simulink model "ctrlSys_rl_env_test"  (R2025b)
settings: Solver=ode14x  StartTime=0.0  StopTime=100  FixedStep=Ts_local  RelTol=1e-4
model workspace (MAT data in the model file):
  CtrlChoice = "MPC_QP"
  FSI_max = [111.58614649; 109.244229433; 111.951462771]
  FSI_min = [3.65502707696; 3.64264743495; 3.42913459589]
  GateChoice = "linear"
  K1 = 1
  K2 = 1e-06
  Ncycle = 25
  SampEn_max = [0.399850516102; 0.373441099122; 0.45958437331]
  SampEn_min = [0.118794892672; 0.117721768048; 0.119599512992]
  fs = 5000
  m = 2
  rRatio = 0.2
values from neighbouring files (symbols this model uses):
  f = 50.0    [ctrlSys.sldd]
  Ts_ctrl = 0.1    [ctrlSys.sldd]
  Ts_local = 1.0E-5    [ctrlSys.sldd]
  Ts_meas = 0.005    [ctrlSys.sldd]
undefined symbols (not defined in the file or in its folder): R_rms, Rn_SNR, Ts_dist, v_lb, v_ub
libraries: ee_lib x13, simulink x5, nesl_utility x4, fl_lib x3, eeRmsMeasurement x3, rllib x1, slpidlib x1
settings Model: DataDictionary=ctrlSys.sldd  SimulationMode=accelerator  Creator=LYG  LastModifiedBy=i336
settings SolverCC: ZeroCrossControl=DisableAll
settings DataIOCC: SaveOutput=off  DSMLogging=off  SaveTime=off  ReturnWorkspaceOutputs=off

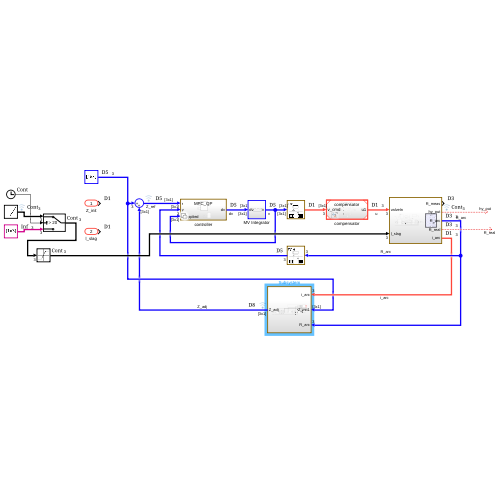
[thumbnail: Simulink's stored preview of the top-level diagram]
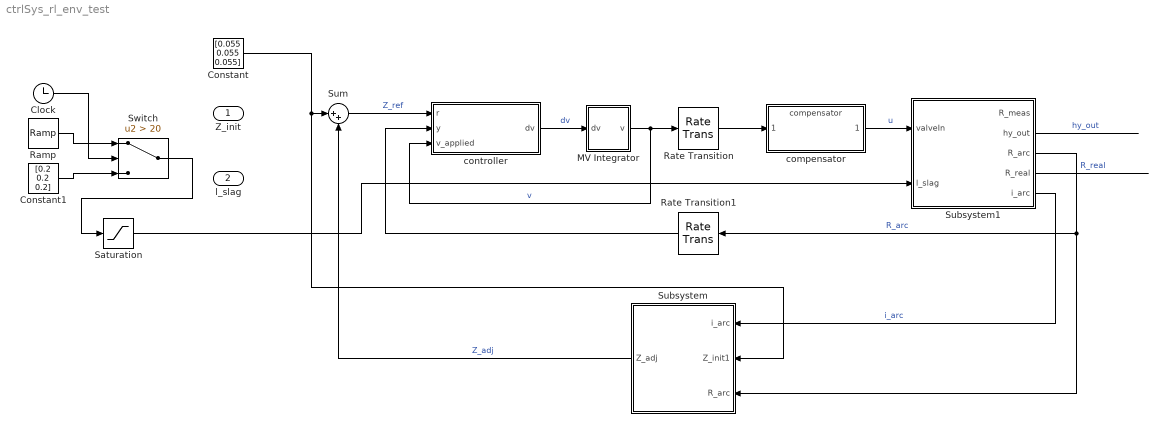
== system ctrlSys_rl_env_test ==
  Z_init : Inport  PortDimensions=3
  l_slag : Inport  Port=2  PortDimensions=3
  Clock : Clock
  Constant : Constant  Value=[0.055 0.055 0.055]  SampleTime=Ts_ctrl
  Constant1 : Constant  Value=[0.2 0.2 0.2]
  MV Integrator : Subsystem
  Ramp : simulink/Sources/Ramp  slope=(0.21 - 0.165) / (600 - 120)  start=[120 120 120]  InitialOutput=0.165
  Rate Transition : RateTransition  OutPortSampleTime=Ts_local
  Rate Transition1 : RateTransition  OutPortSampleTime=Ts_ctrl
  Saturation : Saturate  UpperLimit=0.21  LowerLimit=0
  Subsystem : Subsystem
  Subsystem1 : Subsystem
  Sum : Sum  Inputs=|++
  Switch : Switch  Criteria=u2 > Threshold  Threshold=20  SaturateOnIntegerOverflow=off  InputSameDT=off
  compensator : ModelReference  ModelNameDialog=compensator.slx  SimulationMode=Normal  ModelReferenceVersion=1.24
  controller : Subsystem  Variant=on
  wires:
  Rate Transition/1 -> compensator/1
  compensator/1 -> Subsystem1/1(valveIn)  "u"
  Subsystem1/3(R_arc) -> Subsystem/3(R_arc), Rate Transition1/1  "R_arc"
  Subsystem1/4(R_real) -> ?  "R_real"
  Rate Transition1/1 -> controller/2(y)
  MV Integrator/1(v) -> controller/3(v_applied), Rate Transition/1  "v"
  controller/1(dv) -> MV Integrator/1(dv)  "dv"
  Sum/1 -> controller/1(r)  "Z_ref"
  Subsystem/1(Z_adj) -> Sum/2  "Z_adj"
  Subsystem1/5(i_arc) -> Subsystem/1(i_arc)  "i_arc"
  Subsystem1/2(hy_out) -> ?  "hy_out"
  Constant/1 -> Subsystem/2(Z_init1), Sum/1
  Saturation/1 -> Subsystem1/2(l_slag)
  Clock/1 -> Switch/2
  Ramp/1 -> Switch/1
  Constant1/1 -> Switch/3
  Switch/1 -> Saturation/1

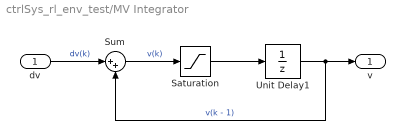
== system ctrlSys_rl_env_test/MV Integrator ==
  dv : Inport
  Saturation : Saturate  UpperLimit=v_ub  LowerLimit=v_lb
  Sum : Sum  Inputs=|++
  Unit Delay1 : UnitDelay  SampleTime=-1  HasFrameUpgradeWarning=on
  v : Outport
  wires:
  Saturation/1 -> Unit Delay1/1
  Unit Delay1/1 -> v/1, Sum/2  "v(k - 1)"
  dv/1 -> Sum/1  "dv(k)"
  Sum/1 -> Saturation/1  "v(k)"

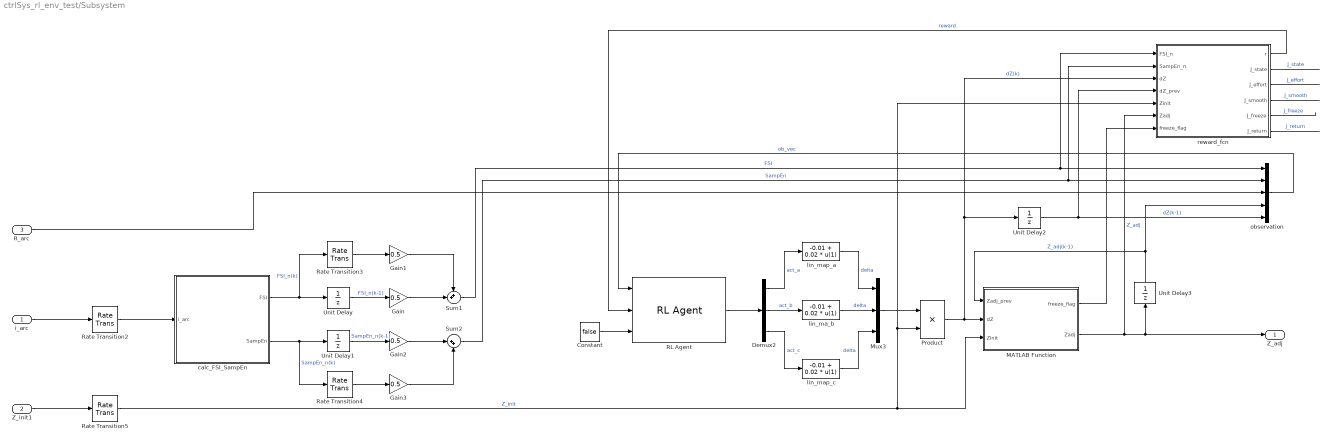
== system ctrlSys_rl_env_test/Subsystem ==
  i_arc : Inport  SampleTime=Ts_local
  Z_init1 : Inport  Port=2  PortDimensions=[3 1]  SampleTime=Ts_ctrl
  R_arc : Inport  Port=3  PortDimensions=3  SampleTime=Ts_meas
  Constant : Constant  Value=false
  Demux2 : Demux  Outputs=3
  Gain{,1..3} (4 alike) : Gain  Gain=0.5
  MATLAB Function : MATLAB Function  TreatAsAtomicUnit=on
  Mux3 : Mux  Inputs=3
  Product : Product
  RL Agent : rllib/RL Agent  Agent=agent  ExternalActionAsInput=off  ProvideLastAction=off  ProvideCumRwd=off  TreatAsDirectFeedthrough=on  UseStrictObservationDataTypes=off
  Rate Transition2 : RateTransition  OutPortSampleTime=1 / fs
  Rate Transition3 : RateTransition  OutPortSampleTime=Ncycle * (1 / f)
  Rate Transition4 : RateTransition  OutPortSampleTime=Ncycle * (1 / f)
  Rate Transition5 : RateTransition  OutPortSampleTime=Ts_sup
  Sum1 : Sum  Inputs=++|
  Sum2 : Sum  Inputs=|++
  Unit Delay : UnitDelay  SampleTime=Ncycle * (1 / f)  HasFrameUpgradeWarning=on
  Unit Delay1 : UnitDelay  SampleTime=Ncycle * (1 / f)  HasFrameUpgradeWarning=on
  Unit Delay2 : UnitDelay  SampleTime=-1  HasFrameUpgradeWarning=on
  Unit Delay3 : UnitDelay  SampleTime=-1  HasFrameUpgradeWarning=on
  calc_FSI_SampEn : MATLAB Function  TreatAsAtomicUnit=on  SystemSampleTime=1 / fs
  lin_ma_b : Fcn  Expr=-0.01 + 0.02 * u(1)
  lin_map_a : Fcn  Expr=-0.01 + 0.02 * u(1)
  lin_map_c : Fcn  Expr=-0.01 + 0.02 * u(1)
  observation : Mux  Inputs=5
  reward_fcn : MATLAB Function  TreatAsAtomicUnit=on
  Z_adj : Outport
  wires:
  Gain2/1 -> Sum2/1
  lin_map_c/1 -> Mux3/3  "delta"
  Z_init1/1 -> Rate Transition5/1
  Rate Transition5/1 -> MATLAB Function/3(Zinit), Product/2, reward_fcn/5(Zinit)  "Z_init"
  Unit Delay1/1 -> Gain2/1  "SampEn_n(k-1)"
  Rate Transition4/1 -> Gain3/1
  Unit Delay2/1 -> reward_fcn/4(dZ_prev), observation/5  "dZ(k-1)"
  calc_FSI_SampEn/1(FSI) -> Rate Transition3/1, Unit Delay/1  "FSI_n(k)"
  Sum2/1 -> reward_fcn/2(SampEn_n), observation/2  "SampEn"
  Demux2/2 -> lin_ma_b/1  "act_b"
  MATLAB Function/2(Zadj) -> reward_fcn/6(Zadj), Z_adj/1, Unit Delay3/1  "Z_adj"
  Product/1 -> MATLAB Function/2(dZ), reward_fcn/3(dZ), Unit Delay2/1  "dZ(k)"
  Demux2/3 -> lin_map_c/1  "act_c"
  lin_map_a/1 -> Mux3/1  "delta"
  Mux3/1 -> Product/1
  Gain3/1 -> Sum2/2
  Constant/1 -> RL Agent/3
  Demux2/1 -> lin_map_a/1  "act_a"
  R_arc/1 -> observation/3
  i_arc/1 -> Rate Transition2/1
  Unit Delay/1 -> Gain/1  "FSI_n(k-1)"
  Rate Transition3/1 -> Gain1/1
  MATLAB Function/1(freeze_flag) -> reward_fcn/7(freeze_flag)
  Gain/1 -> Sum1/2
  Sum1/1 -> reward_fcn/1(FSI_n), observation/1  "FSI"
  Unit Delay3/1 -> observation/4, MATLAB Function/1(Zadj_prev)  "Z_adj(k-1)"
  calc_FSI_SampEn/2(SampEn) -> Rate Transition4/1, Unit Delay1/1  "SampEn_n(k)"
  lin_ma_b/1 -> Mux3/2  "delta"
  Rate Transition2/1 -> calc_FSI_SampEn/1(i_arc)
  Gain1/1 -> Sum1/1
  observation/1 -> RL Agent/1  "ob_vec"
  reward_fcn/1(r) -> RL Agent/2  "reward"
  RL Agent/1 -> Demux2/1
  reward_fcn/2(J_state) -> ?  "J_state"
  reward_fcn/3(J_effort) -> ?  "J_effort"
  reward_fcn/4(J_smooth) -> ?  "J_smooth"
  reward_fcn/5(J_freeze) -> ?  "J_freeze"
  reward_fcn/6(J_return) -> ?  "J_return"

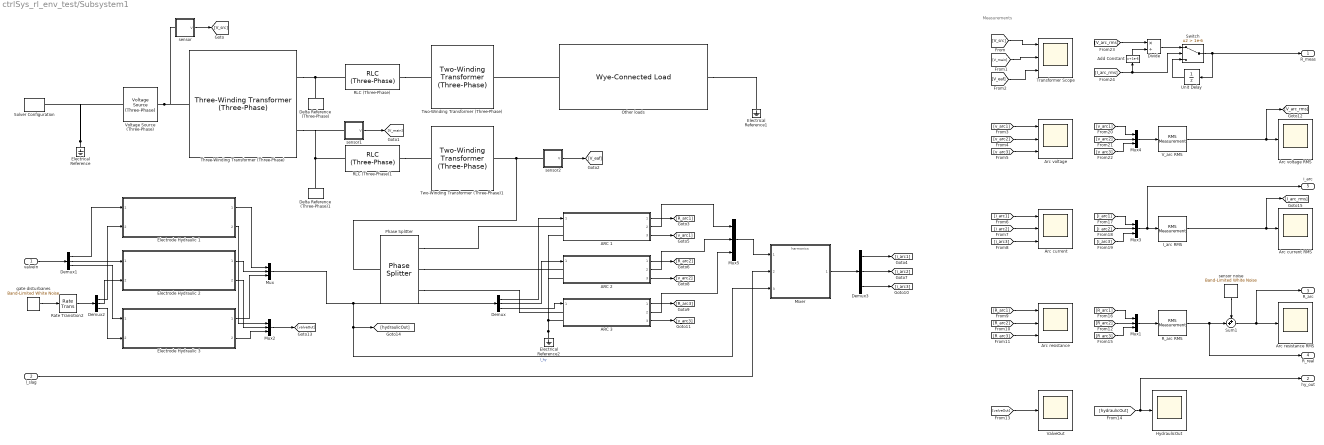
== system ctrlSys_rl_env_test/Subsystem1 ==
  note: Measurements
  valveIn : Inport
  l_slag : Inport  Port=2
  ARC 1 : Subsystem  ReferencedSubsystem=Arc_System
  ARC 2 : Subsystem  ReferencedSubsystem=Arc_System
  ARC 3 : Subsystem  ReferencedSubsystem=Arc_System
  Add Constant : Bias  Bias=1e-6  SaturateOnIntegerOverflow=off
  Arc current : Scope  NumInputPorts=3
      settings: ActiveDisplayYMinimum=-41973.164268779663  ActiveDisplayYMaximum=41974.004776580055  DataLoggingVariableName=ScopeData2
  Arc current RMS : Scope
      settings: ActiveDisplayYMinimum=-3055.4847803654839  ActiveDisplayYMaximum=27499.363023289359  DataLoggingVariableName=ScopeData7
  Arc resistance : Scope  NumInputPorts=3
      settings: ActiveDisplayYMinimum=-0.1125194623785952  ActiveDisplayYMaximum=1.0569916577736953  DataLoggingVariableName=ScopeData3
  Arc resistance RMS : Scope
      settings: ActiveDisplayYMinimum=-0.083534916885155491  ActiveDisplayYMaximum=0.7518142519663995  DataLoggingVariableName=ScopeData4
  Arc voltage : Scope  NumInputPorts=3
      settings: ActiveDisplayYMinimum=351.3925306602107  ActiveDisplayYMaximum=415.43919686304929
  Arc voltage RMS : Scope
      settings: ActiveDisplayYMinimum=-47.465203373542423  ActiveDisplayYMaximum=427.18683036188185  DataLoggingVariableName=ScopeData8
  Delta Reference (Three-Phase) : ee_lib/Connectors & References/Delta Reference (Three-Phase)
      settings: InternalSimscapePortConfiguration="{\"Bottom\":[],\"Left\":[{\"id\":\"N\",\"label\":\"~\",\"type\":\"foundation.electrical.three_phase\"}],\"Right\":[],\"Top\":[]}"
  Delta Reference (Three-Phase)1 : ee_lib/Connectors & References/Delta Reference (Three-Phase)
      settings: InternalSimscapePortConfiguration="{\"Bottom\":[],\"Left\":[{\"id\":\"N\",\"label\":\"~\",\"type\":\"foundation.electrical.three_phase\"}],\"Right\":[],\"Top\":[]}"
  Demux{,1..3} (4 alike) : Demux  Outputs=3
  Divide : Product  Inputs=*/  OutMin=0
  Electrical Reference : fl_lib/Electrical/Electrical Elements/Electrical Reference
  Electrical Reference1 : fl_lib/Electrical/Electrical Elements/Electrical Reference
  Electrical Reference2 : fl_lib/Electrical/Electrical Elements/Electrical Reference
  Electrode Hydraulic 1 : Subsystem  ReferencedSubsystem=Electrode_Hydraulic
  Electrode Hydraulic 2 : Subsystem  ReferencedSubsystem=Electrode_Hydraulic
  Electrode Hydraulic 3 : Subsystem  ReferencedSubsystem=Electrode_Hydraulic
  HydraulicOut : Scope
      settings: ActiveDisplayYMinimum=0.49663037739310889  ActiveDisplayYMaximum=0.6160273324010842  DataLoggingVariableName=ScopeData6
  I_arc RMS : eeRmsMeasurement/RMS Measurement  LabelModeActiveChoice=Total  F=f  SpecifyHarmonics=off  K=[0 1 2]  Ts=Ts_meas
      settings: LibrarySourceBlock=|
      | ee_sl_lib/Measurements/RMS
      | Measurement
  Mixer : ModelReference  ModelNameDialog=harmonics.slx  SimulationMode=Normal  ModelReferenceVersion=1.73
  Mux{,1..5} (6 alike) : Mux  Inputs=3
  Other loads : ee_lib/Passive/RLC Assemblies/Wye-Connected Load  port_option=ee.enum.threePhasePort.composite  parameterization=ee.enum.rlc.parameterization.ratedpower  component_structure=ee.enum.rlc.structure.R  component_structure_PQ=ee.enum.rlc.structure.SeriesRLC  R=1 Ohm  L=1e-3 H  C=1e-6 F  VRated=6000 V  FRated=f Hz  P=10000 W  Qpos=100 A*V  Qneg=-1e2 A*V  R_parasitic=0 Ohm  G_parasitic=0 1/Ohm  R_parasitic_PQ=0 Ohm  G_parasitic_PQ=0 1/Ohm  Vmag0=24e3 V  Vang0=0 deg  Freq0=60 Hz  IL_specify=off  IL_priority=High  IL=[0, 0, 0] A  IL_nominal_specify=off  IL_nominal_value=1  IL_nominal_unit=A  VC_specify=off  VC_priority=High  VC=[0, 0, 0] V  VC_nominal_specify=off  VC_nominal_value=1  VC_nominal_unit=V
  Phase Splitter : ee_lib/Connectors & References/Phase Splitter
  RLC (Three-Phase) : ee_lib/Passive/RLC Assemblies/RLC (Three-Phase)  port_option=ee.enum.threePhasePort.composite  component_structure=ee.enum.rlc.structure.R  R=0.256 Ohm  L=8e-3 H  C=1e-6 F  R_parasitic=0 Ohm  G_parasitic=0 1/Ohm  IL_specify=off  IL_priority=High  IL=[0, 0, 0] A  IL_nominal_specify=off  IL_nominal_value=1  IL_nominal_unit=A  VC_specify=off  VC_priority=High  VC=[0, 0, 0] V  VC_nominal_specify=off  VC_nominal_value=1  VC_nominal_unit=V
      settings: InternalSimscapePortConfiguration="{\"Bottom\":[],\"Left\":[{\"id\":\"N1\",\"label\":\"~1\",\"type\":\"foundation.electrical.three_phase\"}],\"Right\":[{\"id\":\"N2\",\"label\":\"~2\",\"type\":\"foundation.electrical.three_phase\"}],\"Top\":[]}"
  RLC (Three-Phase)1 : ee_lib/Passive/RLC Assemblies/RLC (Three-Phase)  port_option=ee.enum.threePhasePort.composite  component_structure=ee.enum.rlc.structure.R  R=0.256 Ohm  L=8e-3 H  C=1e-6 F  R_parasitic=0 Ohm  G_parasitic=0 1/Ohm  IL_specify=off  IL_priority=High  IL=[0, 0, 0] A  IL_nominal_specify=off  IL_nominal_value=1  IL_nominal_unit=A  VC_specify=off  VC_priority=High  VC=[0, 0, 0] V  VC_nominal_specify=off  VC_nominal_value=1  VC_nominal_unit=V
      settings: InternalSimscapePortConfiguration="{\"Bottom\":[],\"Left\":[{\"id\":\"N1\",\"label\":\"~1\",\"type\":\"foundation.electrical.three_phase\"}],\"Right\":[{\"id\":\"N2\",\"label\":\"~2\",\"type\":\"foundation.electrical.three_phase\"}],\"Top\":[]}"
  R_arc RMS : eeRmsMeasurement/RMS Measurement  LabelModeActiveChoice=Total  F=f  SpecifyHarmonics=off  K=[0 1 2]  Ts=Ts_meas
      settings: LibrarySourceBlock=|
      | ee_sl_lib/Measurements/RMS
      | Measurement
  Rate Transition2 : RateTransition  OutPortSampleTime=Ts_local
  Solver Configuration : nesl_utility/Solver Configuration  PhysicalDomain=network_engine_domain  SubClassName=solver  LeftPortType=input  RightPortType=generic  Tones=[]  Harmonics=[]  SimulateNoise=off  Profile=off  UseLocalSampling=off  EnableSwitchedLinearOptims=on  FrequencyDomain=off  UseCCode=off  RelTol=0.001  AbsTol=0.001  MinStep=1e-09  ToWorkspace=off  RevertToSquareIcSolve=off  NumHomotopyIterations=100  PhasorMode=off  PhasorModeNumHarmonics=1  ConsistencySolver=NEWTON_XTOL_AFTER_FTOL  IndexReductionMethod=DerivativeReplacement  DoDC=off  ResidualTolerance=1e-09  ConsistencyTolSource=GLOBAL  ConsistencyAbsTol=0.001  ConsistencyRelTol=0.001  ConsistencyTolFactor=0.001  UseLocalSolver=on  LocalSolverChoice=NE_BACKWARD_EULER_ADVANCER  ResolveIndetEquations=on  FunctionEvalNumThread=1  LocalSolverSampleTime=Ts_local  DoFixedCost=off  MaxNonlinIter=5  MaxModeIter=2  ComputeImpulses=off  ImpulseIterations=2  LinearAlgebra=auto  LinearAlgebraNumThread=0  EquationFormulation=NE_TIME_EF  DelaysMemoryBudget=1024  AutomaticFiltering=on  FilteringTimeConstant=0.001  PartitionStorageMethod=AS_NEEDED  PartitionMemoryBudget=1024  PartitionMethod=ROBUST  MultibodyUseLocalSolver=off  MultibodyLocalSolverChoice=ODE1  MultibodyLocalSolverSampleTime=0.001
  Sum1 : Sum  Inputs=++|
  Switch : Switch  Criteria=u2 > Threshold  Threshold=1e-6  SaturateOnIntegerOverflow=off  InputSameDT=off
  Three-Winding Transformer (Three-Phase) : ee_lib/Passive/Transformers/Three-Winding Transformer (Three-Phase)  SRated=100e6 A*V  FRated=f Hz  Winding1Connection=ee.enum.windingconnection.delta1  VRated1=110e3 V  Winding2Connection=ee.enum.windingconnection.delta1  VRated2=3.5e3 V  Winding3Connection=ee.enum.windingconnection.delta1  VRated3=3.5e3 V  CoreType=ee.enum.coretype.threelimb  pu_Rw1=0.01  pu_Rw2=0.01  pu_Rw3=0.01  leakage_reactance_option=ee.enum.transformer_leakage.exclude  pu_Xl1=0.05  pu_Xl2=0.05  pu_Xl3=0.05  magnetizing_resistance_option=ee.enum.transformer_magnetizingResistance.exclude  pu_Rm=500  magnetizing_reactance_option=ee.enum.transformer_magnetizingReactance.exclude  saturation_option=ee.enum.transformer_saturation.exclude  pu_Xm=500  current_data=[0, .002, 1, 2]  magnetic_flux_data=[0, 1.2, 1.5, 1.51]  pu_X0=0.5  i1_specify=off  i1_priority=None  i1=[0, 0, 0] A  i1_nominal_specify=off  i1_nominal_value=1  i1_nominal_unit=A  i2_specify=off  i2_priority=None  i2=[0, 0, 0] A  i2_nominal_specify=off  i2_nominal_value=1  i2_nominal_unit=A  i3_specify=off  i3_priority=None  i3=[0, 0, 0] A  i3_nominal_specify=off  i3_nominal_value=1  i3_nominal_unit=A  phi_specify=off  phi_priority=None  phi=[0, 0, 0]  phi_nominal_specify=off  phi_nominal_value=1  phi_nominal_unit=1  power_dissipated_specify=off  power_dissipated_priority=None  power_dissipated=0 W  power_dissipated_nominal_specify=off  power_dissipated_nominal_value=1  power_dissipated_nominal_unit=W
      settings: InternalSimscapePortConfiguration="{\"Bottom\":[],\"Left\":[{\"id\":\"N1\",\"label\":\"~1\",\"type\":\"foundation.electrical.three_phase\"}],\"Right\":[{\"id\":\"N2\",\"label\":\"~2\",\"type\":\"foundation.electrical.three_phase\"},{\"id\":\"N3\",\"label\":\"~3\",\"type\":\"foundation.electrical.three_phase\"}],\"Top\":[]}"
  Transformer Scope : Scope  NumInputPorts=3
      settings: ActiveDisplayYMinimum=-194454.28422245517  ActiveDisplayYMaximum=194453.63939169198
  Two-Winding Transformer (Three-Phase) : ee_lib/Passive/Transformers/Two-Winding Transformer (Three-Phase)  SRated=100e6 A*V  FRated=f Hz  Winding1Connection=ee.enum.windingconnection.delta1  VRated1=735000 V  Winding2Connection=ee.enum.windingconnection.Y  VRated2=8820 V  CoreType=ee.enum.coretype.threelimb  pu_Rw1=0.01  pu_Rw2=0.01  leakage_reactance_option=ee.enum.transformer_leakage.exclude  pu_Xl1=0.05  pu_Xl2=0.05  magnetizing_resistance_option=ee.enum.transformer_magnetizingResistance.exclude  pu_Rm=500  magnetizing_reactance_option=ee.enum.transformer_magnetizingReactance.exclude  saturation_option=ee.enum.transformer_saturation.exclude  pu_Xm=500  current_data=[0, .002, 1, 2]  magnetic_flux_data=[0, 1.2, 1.5, 1.51]  pu_X0=0.5  i1_specify=off  i1_priority=None  i1=[0, 0, 0] A  i1_nominal_specify=off  i1_nominal_value=1  i1_nominal_unit=A  i2_specify=off  i2_priority=None  i2=[0, 0, 0] A  i2_nominal_specify=off  i2_nominal_value=1  i2_nominal_unit=A  phi_specify=off  phi_priority=None  phi=[0, 0, 0]  phi_nominal_specify=off  phi_nominal_value=1  phi_nominal_unit=1  power_dissipated_specify=off  power_dissipated_priority=None  power_dissipated=0 W  power_dissipated_nominal_specify=off  power_dissipated_nominal_value=1  power_dissipated_nominal_unit=W
      settings: InternalSimscapePortConfiguration="{\"Bottom\":[],\"Left\":[{\"id\":\"N1\",\"label\":\"~1\",\"type\":\"foundation.electrical.three_phase\"}],\"Right\":[{\"id\":\"N2\",\"label\":\"~2\",\"type\":\"foundation.electrical.three_phase\"}],\"Top\":[]}"
  Two-Winding Transformer (Three-Phase)1 : ee_lib/Passive/Transformers/Two-Winding Transformer (Three-Phase)  SRated=100e6 A*V  FRated=f Hz  Winding1Connection=ee.enum.windingconnection.delta1  VRated1=3.5e3 V  Winding2Connection=ee.enum.windingconnection.delta1  VRated2=580 V  CoreType=ee.enum.coretype.threelimb  pu_Rw1=0.01  pu_Rw2=0.01  leakage_reactance_option=ee.enum.transformer_leakage.exclude  pu_Xl1=0.05  pu_Xl2=0.05  magnetizing_resistance_option=ee.enum.transformer_magnetizingResistance.exclude  pu_Rm=500  magnetizing_reactance_option=ee.enum.transformer_magnetizingReactance.exclude  saturation_option=ee.enum.transformer_saturation.exclude  pu_Xm=500  current_data=[0, .002, 1, 2]  magnetic_flux_data=[0, 1.2, 1.5, 1.51]  pu_X0=0.5  i1_specify=off  i1_priority=None  i1=[0, 0, 0] A  i1_nominal_specify=off  i1_nominal_value=1  i1_nominal_unit=A  i2_specify=off  i2_priority=None  i2=[0, 0, 0] A  i2_nominal_specify=off  i2_nominal_value=1  i2_nominal_unit=A  phi_specify=off  phi_priority=None  phi=[0, 0, 0]  phi_nominal_specify=off  phi_nominal_value=1  phi_nominal_unit=1  power_dissipated_specify=off  power_dissipated_priority=None  power_dissipated=0 W  power_dissipated_nominal_specify=off  power_dissipated_nominal_value=1  power_dissipated_nominal_unit=W
      settings: InternalSimscapePortConfiguration="{\"Bottom\":[],\"Left\":[{\"id\":\"N1\",\"label\":\"~1\",\"type\":\"foundation.electrical.three_phase\"}],\"Right\":[{\"id\":\"N2\",\"label\":\"~2\",\"type\":\"foundation.electrical.three_phase\"}],\"Top\":[]}"
  Unit Delay : UnitDelay  SampleTime=-1  HasFrameUpgradeWarning=on
  V_arc RMS : eeRmsMeasurement/RMS Measurement  LabelModeActiveChoice=Total  F=f  SpecifyHarmonics=off  K=[0 1 2]  Ts=Ts_meas
      settings: LibrarySourceBlock=|
      | ee_sl_lib/Measurements/RMS
      | Measurement
  ValveOut : Scope
      settings: ActiveDisplayYMinimum=-0.0035141440160345178  ActiveDisplayYMaximum=0.0070571271128927245  DataLoggingVariableName=ScopeData5
  Voltage Source (Three-Phase) : ee_lib/Sources/Voltage Source (Three-Phase)  vline_rms=110e3 V  shift=0 deg  freq=f Hz  impedance_option=0  SShortCircuit=1e6 A*V  XR=15  R=0.01 Ohm  L=3.97e-4 H  harmonic_option=0  harmonic_orders=[5, 7, 11, 13]  harmonic_ratios=[.1, .1, .1, .1]  G_parasitic=0 1/Ohm  I_specify=off  I_priority=None  I=[0, 0, 0] A  I_nominal_specify=off  I_nominal_value=1  I_nominal_unit=A
  gate disturbanes : simulink/Sources/Band-Limited White Noise  Cov=dist_power  Ts=Ts_dist  seed=dist_seed
  sensor : Subsystem
  sensor noise : simulink/Sources/Band-Limited White Noise  Cov=Ts_meas * (R_rms / (10^(Rn_SNR / 20)))^2  Ts=Ts_meas  seed=Rn_seed
  sensor1 : Subsystem
  sensor2 : Subsystem
  R_meas : Outport
  hy_out : Outport  Port=2
  R_arc : Outport  Port=3
  R_real : Outport  Port=4
  i_arc : Outport  Port=5
  wires:
  Electrode Hydraulic 2/1 -> Mux/2
  ARC 2/3 -> [v_arc2]
  Electrode Hydraulic 1/1 -> Mux/1
  [i_arc2] -> Mux3/2
  [V_arc_rms] -> Divide/1
  ARC 3/2 -> Mux5/3
  Demux1/2 -> Electrode Hydraulic 2/1
  [v_arc1] -> Arc voltage/1
  Mux2/1 -> [valveOut]
  Demux3/2 -> [i_arc2]
  [R_arc3] -> Arc resistance/3
  [i_arc1] -> Mux3/1
  Demux3/3 -> [i_arc3]
  [R_arc2] -> Mux1/2
  ARC 2/2 -> Mux5/2
  [v_arc2] -> Mux4/2
  [R_arc3] -> Mux1/3
  gate disturbanes/1 -> Rate Transition2/1
  l_slag/1 -> Mixer/2
  sensor/1(V) -> [V_src]
  sensor1/1(V) -> [V_main]
  ARC 2/1 -> [R_arc2]
  [i_arc3] -> Arc current/3
  [valveOut] -> ValveOut/1
  Mux4/1 -> V_arc RMS/1
  ARC 1/2 -> Mux5/1
  [v_arc1] -> Mux4/1
  Demux2/2 -> Electrode Hydraulic 2/2
  [I_arc_rms] -> Switch/2, Add Constant/1
  Electrode Hydraulic 3/1 -> Mux/3
  Mixer/1 -> Demux3/1
  [v_arc3] -> Arc voltage/3
  Demux2/3 -> Electrode Hydraulic 3/2
  V_arc RMS/1 -> [V_arc_rms], Arc voltage RMS/1
  Demux/2 -> ARC 2/1
  [V_eaf] -> Transformer Scope/3
  I_arc RMS/1 -> [I_arc_rms], Arc current RMS/1
  valveIn/1 -> Demux1/1
  Electrode Hydraulic 1/2 -> Mux2/1
  Demux/3 -> ARC 3/1
  Mux/1 -> Mixer/3, [hydraulicOut], Demux/1  "l_hy"
  Rate Transition2/1 -> Demux2/1
  [V_main] -> Transformer Scope/2
  [R_arc1] -> Mux1/1
  Mux5/1 -> Mixer/1
  R_arc RMS/1 -> R_real/1, Sum1/2
  sensor2/1(V) -> [V_eaf]
  Demux3/1 -> [i_arc1]
  [R_arc2] -> Arc resistance/2
  [i_arc2] -> Arc current/2
  Mux3/1 -> i_arc/1, I_arc RMS/1
  Demux1/3 -> Electrode Hydraulic 3/1
  [v_arc3] -> Mux4/3
  Add Constant/1 -> Divide/2
  [V_src] -> Transformer Scope/1
  Switch/1 -> R_meas/1, Unit Delay/1
  ARC 1/1 -> [R_arc1]
  ARC 1/3 -> [v_arc1]
  Divide/1 -> Switch/1
  Unit Delay/1 -> Switch/3
  Demux1/1 -> Electrode Hydraulic 1/1
  ARC 3/1 -> [R_arc3]
  sensor noise/1 -> Sum1/1
  Sum1/1 -> R_arc/1, Arc resistance RMS/1
  Demux2/1 -> Electrode Hydraulic 1/2
  Demux/1 -> ARC 1/1
  [R_arc1] -> Arc resistance/1
  [i_arc1] -> Arc current/1
  Electrode Hydraulic 2/2 -> Mux2/2
  [v_arc2] -> Arc voltage/2
  Electrode Hydraulic 3/2 -> Mux2/3
  Mux1/1 -> R_arc RMS/1
  [i_arc3] -> Mux3/3
  [hydraulicOut] -> hy_out/1, HydraulicOut/1
  ARC 3/3 -> [v_arc3]
  connections:
  Phase Splitter/LConn1 -- sensor2/LConn1 -- Two-Winding Transformer (Three-Phase)1/RConn1
  Other loads/RConn1 -- Electrical Reference1/LConn1
  RLC (Three-Phase)/RConn1 -- Two-Winding Transformer (Three-Phase)/LConn1
  Phase Splitter/RConn2 -- ARC 2/LConn1
  Delta Reference (Three-Phase)1/LConn1 -- RLC (Three-Phase)1/LConn1 -- Three-Winding Transformer (Three-Phase)/RConn2 -- sensor1/LConn1
  Voltage Source (Three-Phase)/RConn1 -- Three-Winding Transformer (Three-Phase)/LConn1 -- sensor/LConn1
  Electrical Reference2/LConn1 -- ARC 3/LConn2 -- ARC 1/LConn2 -- ARC 2/LConn2
  Phase Splitter/RConn1 -- ARC 1/LConn1
  Other loads/LConn1 -- Two-Winding Transformer (Three-Phase)/RConn1
  RLC (Three-Phase)1/RConn1 -- Two-Winding Transformer (Three-Phase)1/LConn1
  Delta Reference (Three-Phase)/LConn1 -- Three-Winding Transformer (Three-Phase)/RConn1 -- RLC (Three-Phase)/LConn1
  Electrical Reference/LConn1 -- Voltage Source (Three-Phase)/LConn1 -- Solver Configuration/RConn1
  Phase Splitter/RConn3 -- ARC 3/LConn1

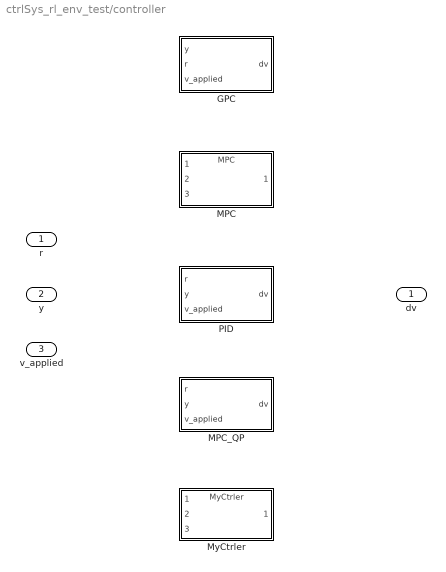
== system ctrlSys_rl_env_test/controller ==
  r : Inport
  y : Inport  Port=2
  v_applied : Inport  Port=3
  GPC : Subsystem  VariantControl="CtrlChoice == \"GPC\""
  MPC : ModelReference  ModelNameDialog=MPC.slx  VariantControl="CtrlChoice == \"MPC\""  ModelReferenceVersion=1.9
  MPC_QP : Subsystem  VariantControl="CtrlChoice == \"MPC_QP\""
  MyCtrler : ModelReference  ModelNameDialog=MyCtrler.slx  SimulationMode=Normal  VariantControl="CtrlChoice == \"MyCtrler\""  ModelReferenceVersion=1.44
  PID : Subsystem  VariantControl="CtrlChoice == \"PID\""
  dv : Outport

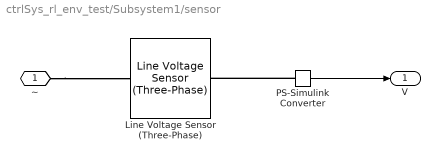
== system ctrlSys_rl_env_test/Subsystem1/sensor ==
  Line Voltage Sensor (Three-Phase) : ee_lib/Sensors & Transducers/Line Voltage Sensor (Three-Phase)
  PS-Simulink Converter : nesl_utility/PS-Simulink Converter  PhysicalDomain=network_engine_domain  SubClassName=ps_output  LeftPortType=input  RightPortType=output  PseudoPeriodic=off  Frequencies=[]  VectorFormat=inherit  Unit=inherit  AffineConversion=off
  ~ : PMIOPort  Side=Left
  V : Outport
  wires:
  PS-Simulink Converter/1 -> V/1
  connections:
  ~/RConn1 -- Line Voltage Sensor (Three-Phase)/LConn1
  PS-Simulink Converter/LConn1 -- Line Voltage Sensor (Three-Phase)/RConn1

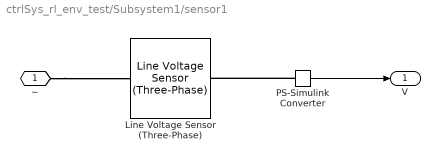
== system ctrlSys_rl_env_test/Subsystem1/sensor1 ==
  Line Voltage Sensor (Three-Phase) : ee_lib/Sensors & Transducers/Line Voltage Sensor (Three-Phase)
  PS-Simulink Converter : nesl_utility/PS-Simulink Converter  PhysicalDomain=network_engine_domain  SubClassName=ps_output  LeftPortType=input  RightPortType=output  PseudoPeriodic=off  Frequencies=[]  VectorFormat=inherit  Unit=inherit  AffineConversion=off
  ~ : PMIOPort  Side=Left
  V : Outport
  wires:
  PS-Simulink Converter/1 -> V/1
  connections:
  ~/RConn1 -- Line Voltage Sensor (Three-Phase)/LConn1
  PS-Simulink Converter/LConn1 -- Line Voltage Sensor (Three-Phase)/RConn1

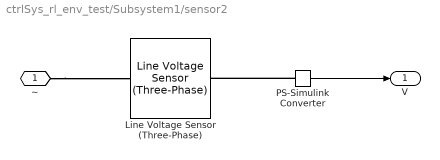
== system ctrlSys_rl_env_test/Subsystem1/sensor2 ==
  Line Voltage Sensor (Three-Phase) : ee_lib/Sensors & Transducers/Line Voltage Sensor (Three-Phase)
  PS-Simulink Converter : nesl_utility/PS-Simulink Converter  PhysicalDomain=network_engine_domain  SubClassName=ps_output  LeftPortType=input  RightPortType=output  PseudoPeriodic=off  Frequencies=[]  VectorFormat=inherit  Unit=inherit  AffineConversion=off
  ~ : PMIOPort  Side=Left
  V : Outport
  wires:
  PS-Simulink Converter/1 -> V/1
  connections:
  PS-Simulink Converter/LConn1 -- Line Voltage Sensor (Three-Phase)/RConn1
  ~/RConn1 -- Line Voltage Sensor (Three-Phase)/LConn1

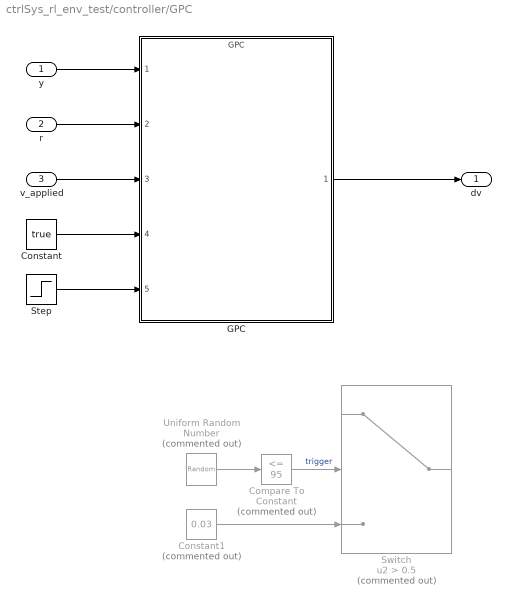
== system ctrlSys_rl_env_test/controller/GPC ==
  y : Inport
  r : Inport  Port=2
  v_applied : Inport  Port=3
  Compare To Constant : simulink/Logic and Bit Operations/Compare To Constant  Commented=on  relop=<=  const=95  OutDataTypeStr=boolean
  Constant : Constant  Value=true
  Constant1 : Constant  Commented=on  Value=0.03  SampleTime=Ts_ctrl
  GPC : ModelReference  ModelNameDialog=GPC.slx  SimulationMode=Normal  ModelReferenceVersion=1.264
  Step : Step  Time=0.1  Before=1  After=0  SampleTime=Ts_ctrl
  Switch : Switch  Commented=on  Criteria=u2 > Threshold  Threshold=0.5  SaturateOnIntegerOverflow=off  InputSameDT=off
  Uniform Random Number : UniformRandomNumber  Commented=on  Minimum=0  Maximum=100  SampleTime=Ts_ctrl * 5
  dv : Outport
  wires:
  v_applied/1 -> GPC/3
  r/1 -> GPC/2
  y/1 -> GPC/1
  Step/1 -> GPC/5
  GPC/1 -> dv/1
  Constant/1 -> GPC/4
  Compare To Constant/1 -> Switch/2  "trigger"
  Uniform Random Number/1 -> Compare To Constant/1
  Constant1/1 -> Switch/3

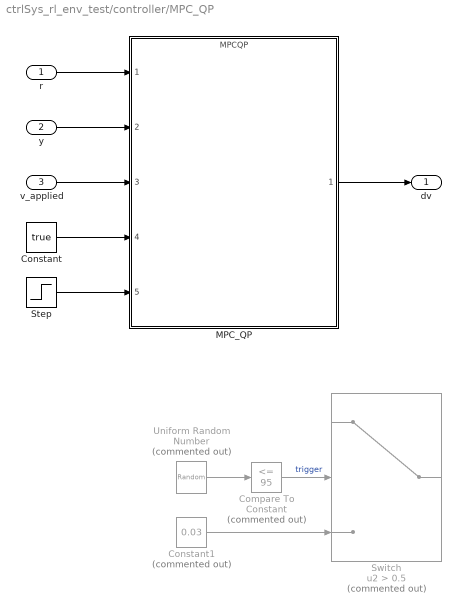
== system ctrlSys_rl_env_test/controller/MPC_QP ==
  r : Inport
  y : Inport  Port=2
  v_applied : Inport  Port=3
  Compare To Constant : simulink/Logic and Bit Operations/Compare To Constant  Commented=on  relop=<=  const=95  OutDataTypeStr=boolean
  Constant : Constant  Value=true
  Constant1 : Constant  Commented=on  Value=0.03  SampleTime=Ts_ctrl
  MPC_QP : ModelReference  ModelNameDialog=MPCQP.slx  SimulationMode=Normal  ModelReferenceVersion=1.61
  Step : Step  Time=0.1  Before=1  After=0  SampleTime=Ts_ctrl
  Switch : Switch  Commented=on  Criteria=u2 > Threshold  Threshold=0.5  SaturateOnIntegerOverflow=off  InputSameDT=off
  Uniform Random Number : UniformRandomNumber  Commented=on  Minimum=0  Maximum=100  SampleTime=Ts_ctrl * 5
  dv : Outport
  wires:
  r/1 -> MPC_QP/1
  v_applied/1 -> MPC_QP/3
  y/1 -> MPC_QP/2
  MPC_QP/1 -> dv/1
  Compare To Constant/1 -> Switch/2  "trigger"
  Uniform Random Number/1 -> Compare To Constant/1
  Constant1/1 -> Switch/3
  Constant/1 -> MPC_QP/4
  Step/1 -> MPC_QP/5

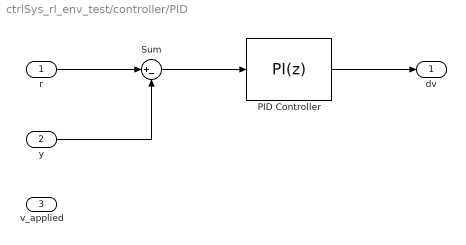
== system ctrlSys_rl_env_test/controller/PID ==
  r : Inport
  y : Inport  Port=2
  v_applied : Inport  Port=3
  PID Controller : slpidlib/PID Controller  Controller=PI  Form=Parallel  TimeDomain=Discrete-time  UseExternalTs=off  SampleTime=Ts_ctrl  IntegratorMethod=Forward Euler  FilterMethod=Forward Euler  ControllerParametersSource=internal  P=100  I=10  UseKiTs=off  D=0  UseExternalDerivativeSource=off  N=100  UseFilter=on  TunerSelectOption=Transfer Function Based (PID Tuner App)  InitialConditionSource=internal  InitialConditionForIntegrator=0  InitialConditionForFilter=0  DifferentiatorICPrevScaledInput=0  ExternalReset=none  TrackingMode=off  Kt=1  LimitOutput=off  SatLimitsSource=internal  UpperSaturationLimit=inf  LowerSaturationLimit=-inf  LinearizeAsGain=on  AntiWindupMode=none  Kb=1  LimitIntegrator=off  UpperIntegratorSaturationLimit=inf  LowerIntegratorSaturationLimit=-inf  POutMin=[]  POutMax=[]  IOutMin=[]  IOutMax=[]  DOutMin=[]  DOutMax=[]  NOutMin=[]  NOutMax=[]  SumOutMin=[]  SumOutMax=[]  SaturationOutMin=[]  SaturationOutMax=[]  PParamMin=[]  PParamMax=[]  IParamMin=[]  IParamMax=[]  DParamMin=[]  DParamMax=[]  NParamMin=[]  NParamMax=[]  KbParamMin=[]  KbParamMax=[]  KtParamMin=[]  KtParamMax=[]  KbOutMin=[]  KbOutMax=[]  KtOutMin=[]  KtOutMax=[]  IntegratorOutMin=[]  IntegratorOutMax=[]  FilterOutMin=[]  FilterOutMax=[]  SumI1OutMin=[]  SumI1OutMax=[]  SumI2OutMin=[]  SumI2OutMax=[]  SumI3OutMin=[]  SumI3OutMax=[]  SumI4OutMin=[]  SumI4OutMax=[]  SumDOutMin=[]  SumDOutMax=[]  DifferentiatorOutMin=[]  DifferentiatorOutMax=[]  FilterDiffOutCoefMin=[]  FilterDiffOutCoefMax=[]  ReciprocalOutMin=[]  ReciprocalOutMax=[]  SumDenOutMin=[]  SumDenOutMax=[]  SumNumOutMin=[]  SumNumOutMax=[]  DivideOutMin=[]  DivideOutMax=[]  UdiffTsProdOutMin=[]  UdiffTsProdOutMax=[]  NTsProdOutMin=[]  NTsProdOutMax=[]  UintegralTsProdOutMin=[]  UintegralTsProdOutMax=[]  UngainTsProdOutMin=[]  UngainTsProdOutMax=[]  ClampingZeroOutDataTypeStr=Inherit: Inherit via back propagation  ClampingZeroOutMin=[]  ClampingZeroOutMax=[]  FilterDenConstantOutDataTypeStr=Inherit: Inherit via back propagation  FilterDenConstantOutMin=[]  FilterDenConstantOutMax=[]  PCopyOutDataTypeStr=Inherit: Inherit via back propagation  PCopyOutMin=[]  PCopyOutMax=[]  NCopyOutDataTypeStr=Inherit: Inherit via back propagation  NCopyOutMin=[]  NCopyOutMax=[]  IntegratorContinuousStateAttributes=''  IntegratorStateMustResolveToSignalObject=off  IntegratorRTWStateStorageClass=Auto  FilterContinuousStateAttributes=''  FilterStateMustResolveToSignalObject=off  FilterRTWStateStorageClass=Auto  ParallelPVariant=InternalParameters  IdealPVariant=Disabled  IVariant=InternalParameters  DVariant=Disabled  IntegratorVariant=Discrete  SatVariant=Disabled  AWVariant=Passthrough  PCopyVariant=Disabled  TRVariant=Disabled  FdbkBlocksVariant=Forward  IdealPFdbkVariant=Disabled  SatFdbkVariant=Disabled  DerivativeFilterVariant=Disabled  NVariant=Disabled  NCopyVariant=Disabled_SignalSpec  FilterICVariant=Disabled  IntegratorICVariant=InternalICs  ExternalResetVariant=Disabled  TRSumVariant=Passthrough  SumFdbkVariant=Disabled  SumVariant=Sum_PI  TsampFilterVariant=InternalTs  TsampNgainVariant=Passthrough  TsampIntegralVariant=Disabled_SignalSpec  ExternalSaturationOutDataTypeStr=Inherit: Same as second input  DerivativeSourceVariant=Disabled  PreIntVariant=InternalPreInt
  Sum : Sum  Inputs=|+-
  dv : Outport
  wires:
  r/1 -> Sum/1
  Sum/1 -> PID Controller/1
  y/1 -> Sum/2
  PID Controller/1 -> dv/1

== matlab function ctrlSys_rl_env_test/Subsystem/reward_fcn ==
  data: FSI_n input; r output; SampEn_n input; dZ input; dZ_prev input; Zinit input; Zadj input; freeze_flag input; J_state output; J_effort output; J_smooth output; J_freeze output; J_return output
function [r, J_state, J_effort, J_smooth, J_freeze, J_return] = RLRewardFcn( ...
    FSI_n, SampEn_n, dZ, dZ_prev, Zinit, Zadj, freeze_flag)
%#codegen
% RL reward for variable-impedance supervisory control
%
% Inputs:
%   FSI_n       : 3x1 normalized FSI in [0,1]
%   SampEn_n    : 3x1 normalized SampEn in [0,1]
%   dZ          : 3x1 current impedance increment (physical value)
%   dZ_prev     : 3x1 previous impedance increment (physical value)
%   Zinit       : 3x1 initial/base impedance
%   Zadj        : 3x1 current adjustable impedance
%   freeze_flag : 3x1, 1 if corresponding phase update is frozen, else 0
%
% Outputs:
%   r           : scalar reward
%   J_state     : state-quality cost
%   J_effort    : control-effort cost
%   J_smooth    : smoothness cost
%   J_freeze    : freeze penalty cost
%   J_return    : return-to-nominal penalty

    % ---------- Hard-coded weights ----------
    alphaF = 1.0;   % weight of FSI term inside state cost
    alphaS = 1.0;   % weight of SampEn term inside state cost

    beta1  = 0.10;  % weight of effort penalty
    % beta2  = 0.20;  % weight of smoothness penalty
    beta2  = 0.0;
    beta3  = 0.50;  % weight of freeze penalty
    % beta4  = 0.30;  % weight of return-to-nominal penalty
    beta4  = 1.0;

    % Buried-arc quality index weights
    wF = 0.5;       % weight of FSI in quality index
    wS = 0.5;       % weight of (1-SampEn) in quality index

    % Smooth gate thresholds:
    % gate = 0 when quality <= G0
    % gate = 1 when quality >= G1
    G0 = 0.75;
    G1 = 0.90;
    % ----------------------------------------

    % Ensure column vectors
    FSI_n       = FSI_n(:);
    SampEn_n    = SampEn_n(:);
    dZ          = dZ(:);
    dZ_prev     = dZ_prev(:);
    Zinit       = Zinit(:);
    Zadj        = Zadj(:);
    freeze_flag = freeze_flag(:);

    % Clamp normalized features to [0,1]
    FSI_n    = min(max(FSI_n, 0.0), 1.0);
    SampEn_n = min(max(SampEn_n, 0.0), 1.0);

    % Safe divisor
    eps_z = 1e-9;
    Zsafe = max(abs(Zinit), eps_z);

    % Normalize dZ to action-like variable in [-1,1]
    % Forward mapping:
    %   dZ = Zinit * (-0.01 + 0.02*a), a in [-1,1]
    % Inverse mapping:
    %   a = (dZ./Zinit + 0.01) / 0.02
    dZ_n      = (dZ      ./ Zsafe + 0.01) / 0.02;
    dZ_prev_n = (dZ_prev ./ Zsafe + 0.01) / 0.02;

    dZ_n      = min(max(dZ_n,      -1.0), 1.0);
    dZ_prev_n = min(max(dZ_prev_n, -1.0), 1.0);

    % Normalize Zadj:
    % allowable range is [-0.1*Zinit, 0], so normalized range is [-1, 0]
    Zadj_n = Zadj ./ (0.1 .* Zsafe);
    Zadj_n = min(max(Zadj_n, -1.0), 0.0);

    % 1) Buried-arc state cost
    % Larger FSI is better, smaller SampEn is better
    J_state = sum(alphaF * (1.0 - FSI_n) + alphaS * SampEn_n);

    % 2) Control-effort cost
    J_effort = sum(dZ_n.^2);

    % 3) Smoothness cost
    J_smooth = sum((dZ_n - dZ_prev_n).^2);

    % 4) Freeze penalty
    J_freeze = sum(freeze_flag ~= 0);

    % 5) Return-to-nominal penalty
    % Quality index: larger means better buried-arc quality
    quality = wF .* FSI_n + wS .* (1.0 - SampEn_n);

    % Smooth gate in [0,1]
    gate = (quality - G0) ./ max(G1 - G0, 1e-9);
    gate = min(max(gate, 0.0), 1.0);

    % Penalize |Zadj| only when buried-arc quality is good
    J_return = sum(gate .* (Zadj_n.^2));

    % Final reward
    r = -J_state ...
        - beta1 * J_effort ...
        - beta2 * J_smooth ...
        - beta3 * J_freeze ...
        - beta4 * J_return;
end

== matlab function ctrlSys_rl_env_test/Subsystem/calc_FSI_SampEn ==
  data: i_arc input size=[3 1]; FSI output; SampEn output; K1 parameter size=[1 1]; K2 parameter size=[1 1]; fs parameter size=[1 1]; Ncycle parameter size=[1 1]; f parameter size=[1 1]; m parameter size=[1 1]; rRatio parameter size=[1 1]; FSI_max parameter size=[3 1]; FSI_min parameter size=[3 1]; SampEn_max parameter size=[3 1]; SampEn_min parameter size=[3 1]
function [FSI, SampEn] = calc_FSI_SampEn( ...
    i_arc, K1, K2, fs, Ncycle, f, m, rRatio, ...
    FSI_max, FSI_min, SampEn_max, SampEn_min)
%#codegen
% i_arc   : 3x1 instantaneous arc current [ia; ib; ic]
% FSI     : 3x1 normalized FSI of three phases
% SampEn  : 3x1 normalized sample entropy of three phases
%
% This version:
% 1) stores samples every call,
% 2) computes features only once every Nhop samples,
% 3) holds the last computed outputs between updates.

    Nwin = int32(Ncycle * fs / f);   % assume exact integer
    Nhop = Nwin;                     % non-overlapping windows
    % For overlapped windows, e.g.:
    % Nhop = int32(Nwin/2);

    persistent buf head count sinceCalc lastFSI lastSampEn

    if isempty(head)
        buf        = zeros(Nwin, 3);
        head       = int32(0);
        count      = int32(0);
        sinceCalc  = int32(0);
        lastFSI    = zeros(3,1);
        lastSampEn = zeros(3,1);
    end

    % Ensure column vector
    i_arc = reshape(i_arc, 3, 1);

    % -------------------------
    % 1) Update circular buffer
    % -------------------------
    head = head + 1;
    if head > Nwin
        head = int32(1);
    end

    buf(head, :) = i_arc.';

    if count < Nwin
        count = count + 1;
    end

    sinceCalc = sinceCalc + 1;

    % Default outputs: hold last values
    FSI    = lastFSI;
    SampEn = lastSampEn;

    % Before first full window, output zeros
    if count < Nwin
        FSI(:)    = 0.0;
        SampEn(:) = 0.0;
        return;
    end

    % -----------------------------------------
    % 2) Only recompute once every Nhop samples
    % -----------------------------------------
    if sinceCalc < Nhop
        return;
    end
    sinceCalc = int32(0);

    % Reconstruct ordered window: oldest --> newest
    xwin = zeros(Nwin, 3);
    if head < Nwin
        n1 = Nwin - head;
        xwin(1:n1, :)      = buf(head+1:Nwin, :);
        xwin(n1+1:Nwin, :) = buf(1:head, :);
    else
        xwin = buf;
    end

    % Compute features phase by phase
    for p = 1:3
        x = xwin(:, p);

        fsi_raw = local_fsi(x, fs, f, K1, K2);
        den1 = FSI_max(p) - FSI_min(p);
        if abs(den1) <= 1e-12
            FSI(p) = 0.0;
        else
            FSI_n = (fsi_raw - FSI_min(p)) / den1;
            FSI(p) = min(max(FSI_n, 0.0), 1.0);
        end

        se_raw = local_sampen(x, m, rRatio);
        den2 = SampEn_max(p) - SampEn_min(p);
        if abs(den2) <= 1e-12
            SampEn(p) = 0.0;
        else
            SampEn_n = (se_raw - SampEn_min(p)) / den2;
            SampEn(p) = min(max(SampEn_n, 0.0), 1.0);
        end
    end

    % Save outputs for holding until next update
    lastFSI    = FSI;
    lastSampEn = SampEn;
end

function y = local_fsi(x, fs, f0, K1, K2)
% Compute FSI from one phase current window

    x = x(:);
    N = length(x);

    % Remove DC component
    x = x - mean(x);

    % FFT
    X = fft(x);

    % Single-sided amplitude spectrum
    nHalf = floor(N/2) + 1;
    A = 2.0 * abs(X(1:nHalf)) / N;
    A(1) = abs(X(1)) / N;
    if mod(N, 2) == 0
        A(end) = abs(X(nHalf)) / N;
    end

    % Extract harmonic amplitudes H1 ... H20
    H = zeros(20, 1);
    for h = 1:20
        k = round(h * f0 / fs * N) + 1;
        if k >= 1 && k <= nHalf
            H(h) = A(k);
        else
            H(h) = 0.0;
        end
    end

    denom = K1 * sqrt(sum(H(10:20).^2)) + K2;

    if denom <= 1e-12
        y = 0.0;
    else
        y = H(1) / denom;
    end
end

function se = local_sampen(x, m, rRatio)
% Compute sample entropy of one phase current window

    x = x(:);
    N = length(x);

    if N <= m + 1
        se = 0.0;
        return;
    end

    sigma = std(x);
    r = rRatio * sigma;

    if r <= 1e-12
        se = 0.0;
        return;
    end

    A = 0.0;
    B = 0.0;

    Nm = N - m;

    for i = 1:Nm
        for j = i+1:Nm
            match_m = true;

            for k = 0:m-1
                if abs(x(i+k) - x(j+k)) > r
                    match_m = false;
                    break;
                end
            end

            if match_m
                B = B + 1.0;

                if abs(x(i+m) - x(j+m)) <= r
                    A = A + 1.0;
                end
            end
        end
    end

    se = -log((A + realmin) / (B + realmin));
end

== matlab function ctrlSys_rl_env_test/Subsystem/MATLAB Function ==
  data: freeze_flag output; Zadj_prev input; Zadj output; dZ input; Zinit input
function [freeze_flag, Zadj] = update_Zadj_with_freeze(Zadj_prev, dZ, Zinit)
%#codegen
% Zadj_prev, dZ, Zinit: 3x1 vectors
% Zadj: updated 3x1 vector
% freeze_flag: 3x1 logical/double vector

    Zadj_prev = Zadj_prev(:);
    dZ        = dZ(:);
    Zinit     = Zinit(:);

    Zcand = Zadj_prev + dZ;
    lower = -0.1 .* Zinit;
    upper = zeros(3,1);

    freeze_flag = (Zcand > upper) | (Zcand < lower);

    Zadj = Zcand;
    Zadj(freeze_flag) = Zadj_prev(freeze_flag);
end
